simulink library "ccsldef"  (R2017a)
settings: Solver=VariableStepAuto  StartTime=0.0  StopTime=10.0  RelTol=1e-3
settings Model: Creator=Li  LastModifiedBy=Li

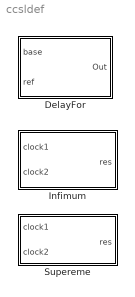
== system ccsldef ==
  DelayFor : Subsystem  TreatAsAtomicUnit=on  mask(DelayFor){delay=0}
      mask help: This block results in a clock by delaying the base clock (base) for a given number of ticks of a reference (ref) clock. The number is given as "delay" parameter.
  "Infimum " : Subsystem  mask(Infimum){}
      mask help: This block generates a clock (res) that is the faster clock between the two clocks (clock1 and clock2).
  Supereme : Subsystem  mask(Supereme){}
      mask help: This block generates a clock (res) that is the slower clock between two clocks (clock1 and clock2).

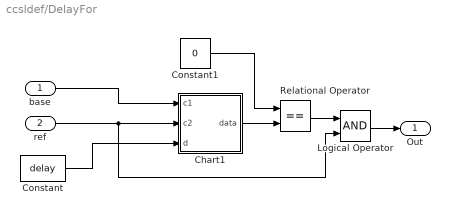
== system ccsldef/DelayFor ==
  base : Inport
  ref : Inport  Port=2
  Chart1 : Stateflow chart  TreatAsAtomicUnit=on
  Constant : Constant  Value=delay
  Constant1 : Constant  Value=0
  Logical Operator : Logic  AllPortsSameDT=off  OutDataTypeStr=boolean
  Relational Operator : RelationalOperator  Operator===  OutDataTypeStr=boolean  RndMeth=Simplest
  Out : Outport
  wires:
  base/1 -> Chart1/1(c1)
  ref/1 -> Logical Operator/2, Chart1/2(c2)
  Constant/1 -> Chart1/3(d)
  Chart1/1(data) -> Relational Operator/2
  Constant1/1 -> Relational Operator/1
  Relational Operator/1 -> Logical Operator/1
  Logical Operator/1 -> Out/1

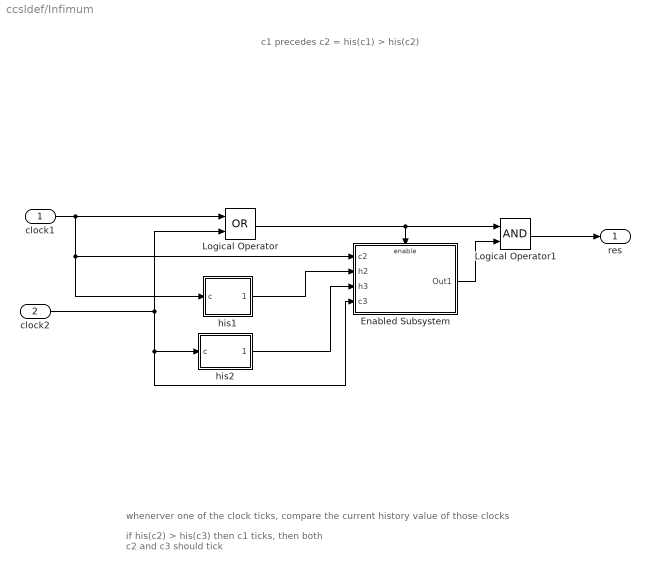
== system ccsldef/Infimum  ==
  note: whenerver one of the clock ticks, compare the current history value of those clocks
  note: if his(c2) > his(c3) then
      | c1 ticks, then both c2 and c3 should tick
  note: c1 precedes c2 = his(c1) > his(c2)
  clock1 : Inport
  clock2 : Inport  Port=2
  Enabled Subsystem : Subsystem  TreatAsAtomicUnit=on
  Logical Operator : Logic  Operator=OR  AllPortsSameDT=off  OutDataTypeStr=boolean
  Logical Operator1 : Logic  AllPortsSameDT=off  OutDataTypeStr=boolean
  his1 : Subsystem
  his2 : Subsystem
  res : Outport
  wires:
  clock1/1 -> Enabled Subsystem/1(c2), his1/1(c), Logical Operator/1
  his1/1(history) -> Enabled Subsystem/2(h2)
  his2/1(history) -> Enabled Subsystem/3(h3)
  Enabled Subsystem/1(Out1) -> Logical Operator1/2
  Logical Operator/1 -> Logical Operator1/1, Enabled Subsystem/Enable
  Logical Operator1/1 -> res/1
  clock2/1 -> Enabled Subsystem/4(c3), his2/1(c), Logical Operator/2

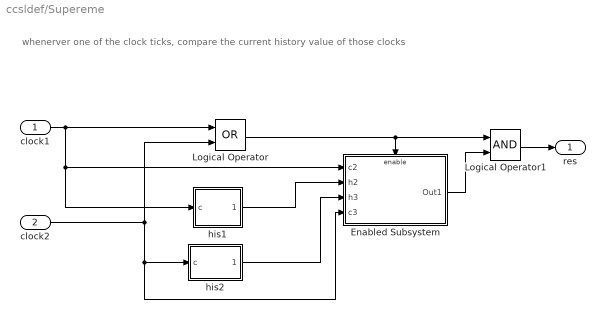
== system ccsldef/Supereme ==
  note: whenerver one of the clock ticks, compare the current history value of those clocks
  clock1 : Inport
  clock2 : Inport  Port=2
  Enabled Subsystem : Subsystem  TreatAsAtomicUnit=on
  Logical Operator : Logic  Operator=OR  AllPortsSameDT=off  OutDataTypeStr=boolean
  Logical Operator1 : Logic  AllPortsSameDT=off  OutDataTypeStr=boolean
  his1 : Subsystem
  his2 : Subsystem
  res : Outport
  wires:
  clock2/1 -> Logical Operator/2, his2/1(c), Enabled Subsystem/4(c3)
  Logical Operator1/1 -> res/1
  Logical Operator/1 -> Enabled Subsystem/Enable, Logical Operator1/1
  Enabled Subsystem/1(Out1) -> Logical Operator1/2
  his2/1(history) -> Enabled Subsystem/3(h3)
  his1/1(history) -> Enabled Subsystem/2(h2)
  clock1/1 -> Logical Operator/1, his1/1(c), Enabled Subsystem/1(c2)

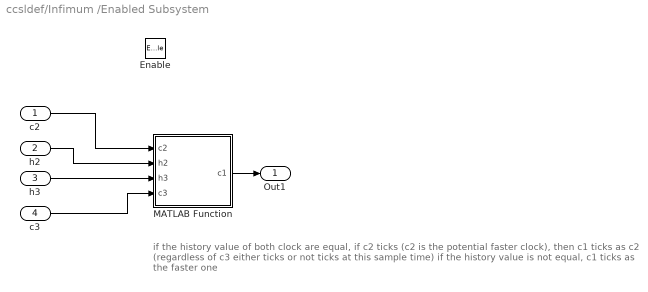
== system ccsldef/Infimum /Enabled Subsystem ==
  note: if the history value of both clock are equal,
      | if c2 ticks (c2 is the potential faster clock), then c1  ticks as c2 (regardless of c3 either ticks or not ticks at this sample time)
      | if the history value is not equal, c1 ticks as the faster one
  c2 : Inport
  h2 : Inport  Port=2
  h3 : Inport  Port=3
  c3 : Inport  Port=4
  Enable : EnablePort
  MATLAB Function : MATLAB Function  TreatAsAtomicUnit=on
  Out1 : Outport
  wires:
  c2/1 -> MATLAB Function/1(c2)
  h2/1 -> MATLAB Function/2(h2)
  h3/1 -> MATLAB Function/3(h3)
  c3/1 -> MATLAB Function/4(c3)
  MATLAB Function/1(c1) -> Out1/1

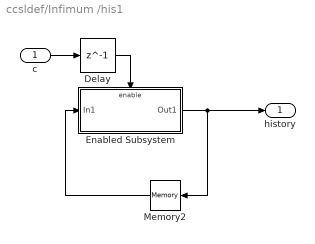
== system ccsldef/Infimum /his1 ==
  c : Inport
  Delay : Delay  DelayLength=1  InitialCondition=0
  Enabled Subsystem : Subsystem  TreatAsAtomicUnit=on
  Memory2 : Memory
  history : Outport
  wires:
  c/1 -> Delay/1
  Delay/1 -> Enabled Subsystem/Enable
  Enabled Subsystem/1(Out1) -> history/1, Memory2/1
  Memory2/1 -> Enabled Subsystem/1(In1)

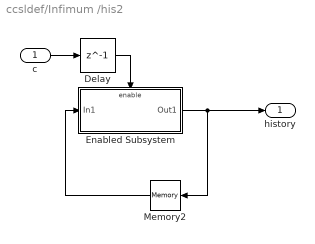
== system ccsldef/Infimum /his2 ==
  c : Inport
  Delay : Delay  DelayLength=1  InitialCondition=0
  Enabled Subsystem : Subsystem  TreatAsAtomicUnit=on
  Memory2 : Memory
  history : Outport
  wires:
  c/1 -> Delay/1
  Delay/1 -> Enabled Subsystem/Enable
  Enabled Subsystem/1(Out1) -> history/1, Memory2/1
  Memory2/1 -> Enabled Subsystem/1(In1)

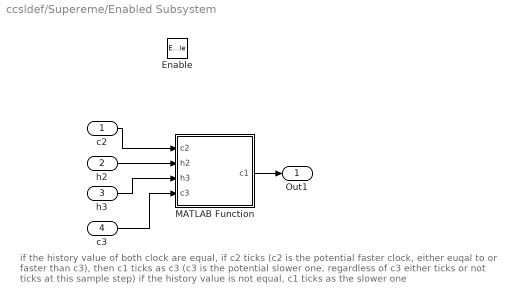
== system ccsldef/Supereme/Enabled Subsystem ==
  note: if the history value of both clock are equal,
      | if c2 ticks (c2 is the potential faster clock, either euqal to or faster than c3), then c1  ticks as c3 (c3 is the potential slower one, regardless of c3 either ticks or not ticks at this sample step)
      | if the history value is not equal, c1 ticks as the slower one
  c2 : Inport
  h2 : Inport  Port=2
  h3 : Inport  Port=3
  c3 : Inport  Port=4
  Enable : EnablePort
  MATLAB Function : MATLAB Function  TreatAsAtomicUnit=on
  Out1 : Outport
  wires:
  MATLAB Function/1(c1) -> Out1/1
  c3/1 -> MATLAB Function/4(c3)
  h3/1 -> MATLAB Function/3(h3)
  h2/1 -> MATLAB Function/2(h2)
  c2/1 -> MATLAB Function/1(c2)

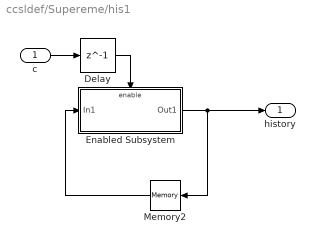
== system ccsldef/Supereme/his1 ==
  c : Inport
  Delay : Delay  DelayLength=1  InitialCondition=0
  Enabled Subsystem : Subsystem  TreatAsAtomicUnit=on
  Memory2 : Memory
  history : Outport
  wires:
  Memory2/1 -> Enabled Subsystem/1(In1)
  Enabled Subsystem/1(Out1) -> Memory2/1, history/1
  Delay/1 -> Enabled Subsystem/Enable
  c/1 -> Delay/1

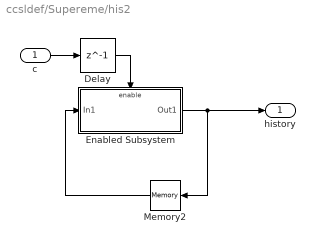
== system ccsldef/Supereme/his2 ==
  c : Inport
  Delay : Delay  DelayLength=1  InitialCondition=0
  Enabled Subsystem : Subsystem  TreatAsAtomicUnit=on
  Memory2 : Memory
  history : Outport
  wires:
  Memory2/1 -> Enabled Subsystem/1(In1)
  Enabled Subsystem/1(Out1) -> Memory2/1, history/1
  Delay/1 -> Enabled Subsystem/Enable
  c/1 -> Delay/1

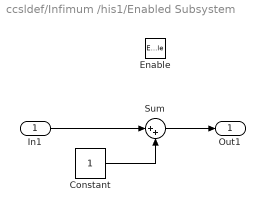
== system ccsldef/Infimum /his1/Enabled Subsystem ==
  In1 : Inport
  Enable : EnablePort
  Constant : Constant
  Sum : Sum  Inputs=|++
  Out1 : Outport
  wires:
  In1/1 -> Sum/1
  Constant/1 -> Sum/2
  Sum/1 -> Out1/1

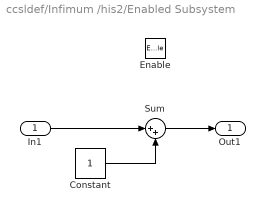
== system ccsldef/Infimum /his2/Enabled Subsystem ==
  In1 : Inport
  Enable : EnablePort
  Constant : Constant
  Sum : Sum  Inputs=|++
  Out1 : Outport
  wires:
  In1/1 -> Sum/1
  Constant/1 -> Sum/2
  Sum/1 -> Out1/1

== system ccsldef/Supereme/his1/Enabled Subsystem ==
  In1 : Inport
  Enable : EnablePort
  Constant : Constant
  Sum : Sum  Inputs=|++
  Out1 : Outport
  wires:
  Sum/1 -> Out1/1
  Constant/1 -> Sum/2
  In1/1 -> Sum/1

== system ccsldef/Supereme/his2/Enabled Subsystem ==
  In1 : Inport
  Enable : EnablePort
  Constant : Constant
  Sum : Sum  Inputs=|++
  Out1 : Outport
  wires:
  Sum/1 -> Out1/1
  Constant/1 -> Sum/2
  In1/1 -> Sum/1

== matlab function ccsldef/Supereme/Enabled Subsystem/MATLAB Function ==
  data: c2 input; c1 output; h2 input; h3 input; c3 input
function c1 = sup(c2, h2, h3, c3)
if h2==h3
    if c2 == 1 % c2 ticks
        c1=c3;
    else       % c3 ticks
        c1=c2;
    end
elseif h2<h3 % c2 runs slower
    c1=c2;
else        % c3 runs slower
    c1=c3;
end

== matlab function ccsldef/Infimum /Enabled Subsystem/MATLAB Function ==
  data: c2 input; c1 output; h2 input; h3 input; c3 input
function c1 = inf(c2, h2, h3, c3)
if h2==h3
    if c2 == 1 % c2 ticks
        c1=c2;
    else       % c3 ticks
        c1=c3;
    end
elseif h2>h3 % c2 runs faster
    c1=c2;
else        % c3 runs faster
    c1=c3;
end

== stateflow chart ccsldef/DelayFor/Chart1 ==
  state exe [parallel]
    en:len=0, Q = -1*ones(1,10), data = -1, test;
    du: test, data=Q(1);
    settings: executionOrder=1
  (default) -> exe
  data: c1 input; c2 input; len local size=1; data output; Q local; T local; d input
  function test:
    | function test
    | % use a queue to count the delayed ticks of c2
    | % if the head of the queue is 0, pop the head
    | if Q(1) == 0
    |     for i = 2:1:len+1 %queue forward by 1
    |     Q(i-1) = Q(i); 
    |     end
    |     len = len - 1;
    | end
    | 
    | % if c1 ticks, then push a new number to count the delayed ticks of c2;
    | if c1 == 1
    |    len = len + 1; %extend the queue
    |    Q(len) = d+1;
    | end
    | 
    | % if c2 ticks, update all the number of ticks in the queue
    | if c2 == 1 
    | for i = 1:1:len
    |     Q(i) = Q(i)-1;
    | end
    | end
    | 
    | end
